simulink model "BlockDiagram"  (Simulink 7.7)
settings: Solver=ode3  StartTime=0.0  StopTime=100  FixedStep=1  RelTol=1e-3
settings Model: Creator=dou1986  LastModifiedBy=kevin
settings DataIOCC: ExternalInput=[t, x]  LoadExternalInput=on  SignalLogging=off
settings DebuggingCC: StrictBusMsg=Warning

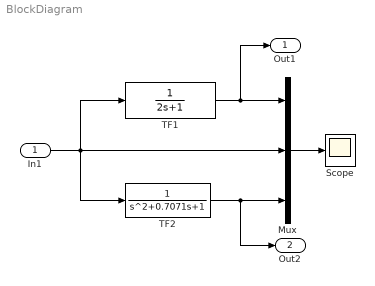
== system BlockDiagram ==
  In1 : Inport
  Mux : Mux  Inputs=3
  Scope : Scope
      settings: TimeRange=100
  TF1 : TransferFcn  Denominator=[2 1]
  TF2 : TransferFcn  Denominator=[1 0.7071 1]
  Out1 : Outport
  Out2 : Outport  Port=2
  wires:
  In1/1 -> TF1/1, TF2/1, Mux/2
  TF1/1 -> Mux/1, Out1/1
  TF2/1 -> Mux/3, Out2/1
  Mux/1 -> Scope/1
